simulink model "project_tank_in_series"  (R2019b)
settings: Solver=FixedStepAuto  StartTime=0.0  StopTime=200  RelTol=1e-3
values from neighbouring files (symbols this model uses):
  C = 2.4    [heated_tank_in_series.m]
  q1 = 10    [heated_tank_in_series.m]
  q2 = 10    [heated_tank_in_series.m]
  q2_1 = -2    [heated_tank_in_series.m]
  q2_2 = +2    (= 2)    [heated_tank_in_series.m]
  q2_3 = +2    (= 2)    [heated_tank_in_series.m]
  q2_4 = -2    [heated_tank_in_series.m]
  q_out = q1+q2    (= 20)    [heated_tank_in_series.m]
  rho = 1000    [heated_tank_in_series.m]
  t1 = 30    [heated_tank_in_series.m]
  T1_0 = 4    [heated_tank_in_series.m]
  T1_1 = -0.5    [heated_tank_in_series.m]
  T1_2 = +0.5    (= 0.5)    [heated_tank_in_series.m]
  T1_3 = +0.5    (= 0.5)    [heated_tank_in_series.m]
  T1_4 = -0.5    [heated_tank_in_series.m]
  T2 = 6    [heated_tank_in_series.m]
  t2 = 60    [heated_tank_in_series.m]
  t3 = 90    [heated_tank_in_series.m]
  T3_0 = (((q1*T1_0/V) + (q2*T2/V)))*(V/q_out)    (= 5)    [heated_tank_in_series.m]
  t4 = 120    [heated_tank_in_series.m]
  T4_0 = double(solve(T4_eq, T4_0))    [heated_tank_in_series.m]
  Th_0 = 152.5    [heated_tank_in_series.m]
  Th_1 = -5    [heated_tank_in_series.m]
  Th_2 = +5    (= 5)    [heated_tank_in_series.m]
  Th_3 = +5    (= 5)    [heated_tank_in_series.m]
  Th_4 = -5    [heated_tank_in_series.m]
  UA = 10000    [heated_tank_in_series.m]
  V = 100    [heated_tank_in_series.m]
libraries: cstblocks x1
settings Model: Creator=oasys  LastModifiedBy=oasys

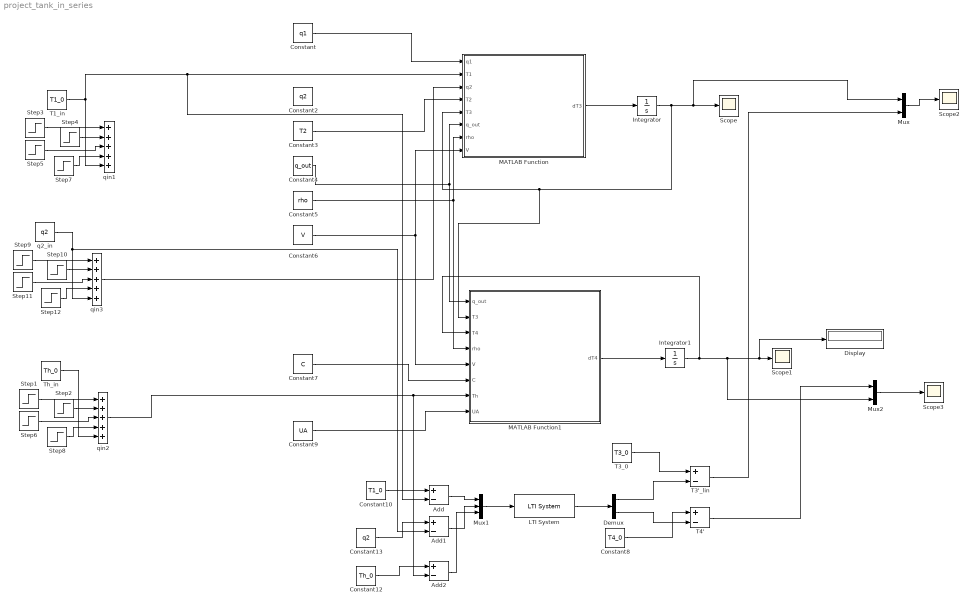
== system project_tank_in_series ==
  Add : Sum  Inputs=+-
  Add1 : Sum  Inputs=+-
  Add2 : Sum  Inputs=+-
  Constant : Constant  Value=q1
  Constant10 : Constant  Value=T1_0
  Constant12 : Constant  Value=Th_0
  Constant13 : Constant  Value=q2
  Constant2 : Constant  Value=q2
  Constant3 : Constant  Value=T2
  Constant4 : Constant  Value=q_out
  Constant5 : Constant  Value=rho
  Constant6 : Constant  Value=V
  Constant7 : Constant  Value=C
  Constant8 : Constant  Value=T4_0
  Constant9 : Constant  Value=UA
  Demux : Demux  Outputs=2
  Display : Display
  Integrator : Integrator  InitialCondition=T1_0
  Integrator1 : Integrator  InitialCondition=T4_0
  LTI System : cstblocks/LTI System  sys=model_lin  IC=[]
  MATLAB Function : MATLAB Function  TreatAsAtomicUnit=on
  MATLAB Function1 : MATLAB Function  TreatAsAtomicUnit=on
  Mux : Mux  Inputs=2
  Mux1 : Mux  Inputs=3
  Mux2 : Mux  Inputs=2
  Scope{,1..3} (4 alike) : Scope
  Step1 : Step  Time=t1  After=Th_1  SampleTime=0
  Step10 : Step  Time=t2  After=q2_2  SampleTime=0
  Step11 : Step  Time=t3  After=q2_3  SampleTime=0
  Step12 : Step  Time=t4  After=q2_4  SampleTime=0
  Step2 : Step  Time=t2  After=Th_2  SampleTime=0
  Step3 : Step  Time=t1  After=T1_1  SampleTime=0
  Step4 : Step  Time=t2  After=T1_2  SampleTime=0
  Step5 : Step  Time=t3  After=T1_3  SampleTime=0
  Step6 : Step  Time=t3  After=Th_3  SampleTime=0
  Step7 : Step  Time=t4  After=T1_4  SampleTime=0
  Step8 : Step  Time=t4  After=Th_4  SampleTime=0
  Step9 : Step  Time=t1  After=q2_1  SampleTime=0
  T1_in : Constant  Value=T1_0
  T3'_lin : Sum  Inputs=+-
  T3_0 : Constant  Value=T3_0
  T4' : Sum  Inputs=+-
  Th_in : Constant  Value=Th_0
  q2_in : Constant  Value=q2
  qin1 : Sum  Inputs=+++++
  qin2 : Sum  Inputs=+++++
  qin3 : Sum  Inputs=+++++
  wires:
  Constant3/1 -> MATLAB Function/4(T2)
  Constant4/1 -> MATLAB Function/6(q_out), MATLAB Function1/1(q_out)
  MATLAB Function/1(dT3) -> Integrator/1
  Integrator/1 -> Mux/1, Scope/1, MATLAB Function/5(T3), MATLAB Function1/2(T3)
  MATLAB Function1/1(dT4) -> Integrator1/1
  Integrator1/1 -> Mux2/2, Display/1, Scope1/1, MATLAB Function1/3(T4)
  Constant5/1 -> MATLAB Function1/4(rho), MATLAB Function/7(rho)
  Constant6/1 -> MATLAB Function/8(V), MATLAB Function1/5(V)
  Constant7/1 -> MATLAB Function1/6(C)
  Constant9/1 -> MATLAB Function1/8(UA)
  Mux/1 -> Scope2/1
  Constant/1 -> MATLAB Function/1(q1)
  Mux1/1 -> LTI System/1
  LTI System/1 -> Demux/1
  Demux/1 -> T3'_lin/2
  Demux/2 -> T4'/2
  T3_0/1 -> T3'_lin/1
  Constant8/1 -> T4'/1
  Mux2/1 -> Scope3/1
  Add/1 -> Mux1/1
  Constant10/1 -> Add/1
  Add1/1 -> Mux1/2
  Constant13/1 -> Add1/1
  Constant12/1 -> Add2/1
  Add2/1 -> Mux1/3
  T4'/1 -> Mux2/1
  T3'_lin/1 -> Mux/2
  Step5/1 -> qin1/3
  Step3/1 -> qin1/1
  T1_in/1 -> qin1/5, Add/2, MATLAB Function/2(T1)
  Step4/1 -> qin1/2
  Step7/1 -> qin1/4
  Step2/1 -> qin2/2
  Step8/1 -> qin2/4
  Step6/1 -> qin2/3
  Th_in/1 -> qin2/5
  Step1/1 -> qin2/1
  Step10/1 -> qin3/2
  Step12/1 -> qin3/4
  Step11/1 -> qin3/3
  q2_in/1 -> Add1/2, qin3/5
  Step9/1 -> qin3/1
  qin2/1 -> Add2/2, MATLAB Function1/7(Th)
  qin3/1 -> MATLAB Function/3(q2)

== matlab function project_tank_in_series/MATLAB Function1 ==
  data: q_out input; dT4 output; T3 input; T4 input; rho input; V input; C input; Th input; UA input
function dT4 = T4(q_out,T3,T4,rho,V,C,Th,UA)
Q = UA*(Th-T4);
dT4 =(q_out*rho*C*(T3 - T4) + Q)/(rho*V*C);

== matlab function project_tank_in_series/MATLAB Function ==
  data: q1 input; dT3 output; T1 input; q2 input; T2 input; T3 input; q_out input; rho input; V input
function dT3 = T3(q1,T1,q2,T2,T3,q_out,rho,V)

dT3 = (T1*q1*rho + T2*q2*rho - T3*q_out*rho)/(rho*V);
